simulink model "TC_SIM"  (R2025b)
settings: Solver=VariableStepAuto  StartTime=0.0  StopTime=10.0  RelTol=1e-12
values from neighbouring files (symbols this model uses):
  A = 1    [PARAMS.m]    (also in PARAMS_IDEAL_LAUNCH_TABLE.m; PID_TUNER.m)
  Cd = 1    [PARAMS.m]    (also in PARAMS_IDEAL_LAUNCH_TABLE.m; PID_TUNER.m)
  cg_f = 0.734568    [PARAMS.m]    (also in PARAMS_IDEAL_LAUNCH_TABLE.m; PID_TUNER.m)
  Cl = 3.8    [PARAMS.m]    (also in PARAMS_IDEAL_LAUNCH_TABLE.m; PID_TUNER.m)
  D = 0    [PID_TUNER.m]
  fd = 4.5    [PARAMS.m]    (also in PARAMS_IDEAL_LAUNCH_TABLE.m; PID_TUNER.m)
  gravity = 9.80665    [PARAMS.m]    (also in PARAMS_IDEAL_LAUNCH_TABLE.m; PID_TUNER.m)
  Grip_Fact = 1.0    (= 1)    [PARAMS.m]    (also in PARAMS_IDEAL_LAUNCH_TABLE.m; PID_TUNER.m)
  h_cg = 0.25273    [PARAMS.m]    (also in PARAMS_IDEAL_LAUNCH_TABLE.m; PID_TUNER.m)
  J = 0.51151    [PARAMS.m]    (also in PARAMS_IDEAL_LAUNCH_TABLE.m; PID_TUNER.m = 1.2)
  Max_Wheel_Omega = (Max_Motor_RPM * 2*pi/60) / fd    (= 162.897396853)    [PARAMS.m]    (also in PARAMS_IDEAL_LAUNCH_TABLE.m; PID_TUNER.m = 183.3)
  Mv = 285.763    [PARAMS.m]    (also in PARAMS_IDEAL_LAUNCH_TABLE.m; PID_TUNER.m)
  r = 0.203    [PARAMS.m]    (also in PARAMS_IDEAL_LAUNCH_TABLE.m; PID_TUNER.m)
  rho = 1.225    [PARAMS.m]    (also in PARAMS_IDEAL_LAUNCH_TABLE.m; PID_TUNER.m)
  Slip_Target = 0.13    [PARAMS.m]    (also in PARAMS_IDEAL_LAUNCH_TABLE.m; PID_TUNER.m)
  T_request = 150    [PARAMS.m]    (also in PARAMS_IDEAL_LAUNCH_TABLE.m; PID_TUNER.m)
  W = 1.53035    [PARAMS.m]    (also in PARAMS_IDEAL_LAUNCH_TABLE.m; PID_TUNER.m)
undefined symbols (not defined in the file or in its folder): I, N, P
libraries: slpidlib x1, simulink x1
settings Model: Creator=jacks  LastModifiedBy=jacks
settings SolverCC: ZeroCrossAlgorithm=Adaptive
settings HardwareCC: ProdHWDeviceType=AMD->x86-64 (Windows64)

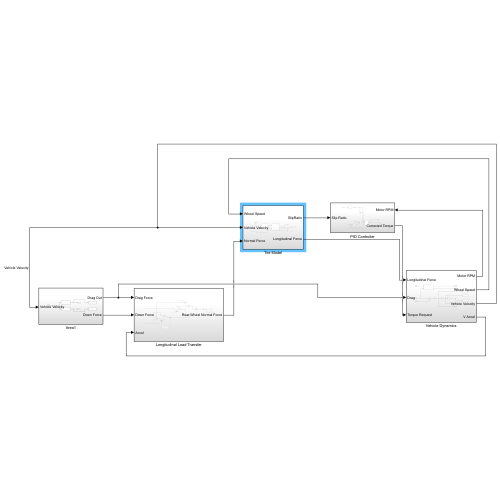
[thumbnail: Simulink's stored preview of the top-level diagram]
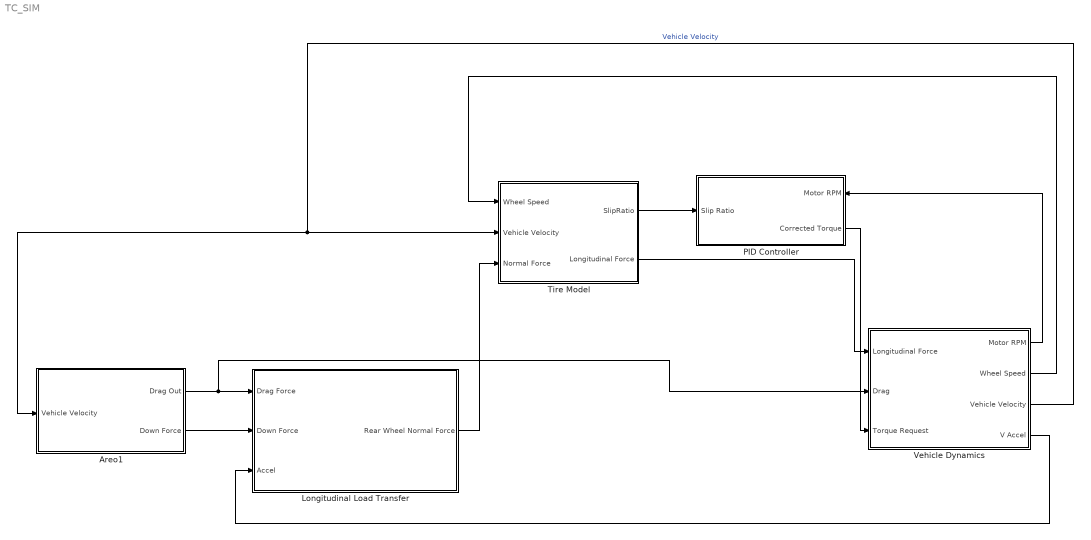
== system TC_SIM ==
  Areo1 : Subsystem
  Longitudinal Load Transfer : Subsystem
  PID Controller : Subsystem
      settings: PortSchema="{\"entries\":[{\"content\":{\"sides\":[{\"content\":{\"connectorIds\":[\"In1\"]},\"type\":\"ConnectorPlacement.EquallySpacedRectSide\",\"uuid\":\"e08c6440-e916-4e80-a3d1-0d9259b5e071\"},{\"content\":{\"connectorIds\":[\"In2\",\"Out1\"],\"side\":\"RIGHT\"},\"type\":\"ConnectorPlacement.EquallySpacedRectSide\",\"uuid\":\"5e4d30b8-f711-4660-8ae3-898fb6763926\"},{\"content\":{\"side\":\"TOP\"},\"type\":\"ConnectorPlacement.EquallySpacedRectSide\",\"uuid\":\"1af7cd33-4532-4fa2-87e1-a13d52e6b401\"}]},\"type\":\"ConnectorPlacement.EquallySpacedConnector\",\"uuid\":\"29b0d2b6-0aba-458c-9448-89d85d2daafa\"}],\"packageUris\":[\"http://schema.mathworks.com/mf0/Connector/R2020b\"],\"version\":\"1.0\"}"
  Tire Model : Subsystem
  Vehicle Dynamics : Subsystem
  wires:
  Vehicle Dynamics/3(Vehicle Velocity) -> Tire Model/2(Vehicle Velocity), Areo1/1(Vehicle Velocity)  "Vehicle Velocity"
  Tire Model/1(SlipRatio) -> PID Controller/1(Slip Ratio)
  Areo1/2(Down Force) -> Longitudinal Load Transfer/2(Down Force)
  Areo1/1(Drag Out) -> Longitudinal Load Transfer/1(Drag Force), Vehicle Dynamics/2(Drag)
  Vehicle Dynamics/4(V Accel) -> Longitudinal Load Transfer/3(Accel)
  Longitudinal Load Transfer/1(Rear Wheel Normal Force) -> Tire Model/3("Normal Force ")
  Tire Model/2(Longitudinal Force) -> Vehicle Dynamics/1(Longitudinal Force)
  Vehicle Dynamics/2(Wheel Speed) -> Tire Model/1(Wheel Speed)
  Vehicle Dynamics/1(Motor RPM) -> PID Controller/2(Motor RPM)
  PID Controller/1(Corrected Torque) -> Vehicle Dynamics/3(Torque Request)

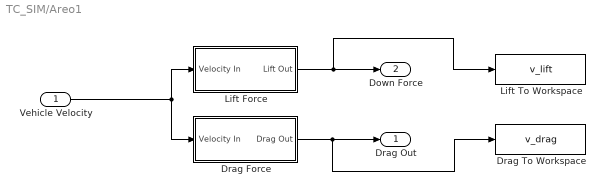
== system TC_SIM/Areo1 ==
  Vehicle Velocity : Inport
  Drag Force : Subsystem
  Drag To Workspace : ToWorkspace  VariableName=v_drag  SaveFormat=Timeseries  SampleTime=-1
  Lift Force : Subsystem
  Lift To Workspace : ToWorkspace  VariableName=v_lift  SaveFormat=Timeseries  SampleTime=-1
  Drag Out : Outport
  Down Force : Outport  Port=2
  wires:
  Lift Force/1(Lift Out) -> Lift To Workspace/1, Down Force/1
  Vehicle Velocity/1 -> Drag Force/1(Velocity In), Lift Force/1(Velocity In)
  Drag Force/1(Drag Out) -> Drag To Workspace/1, Drag Out/1

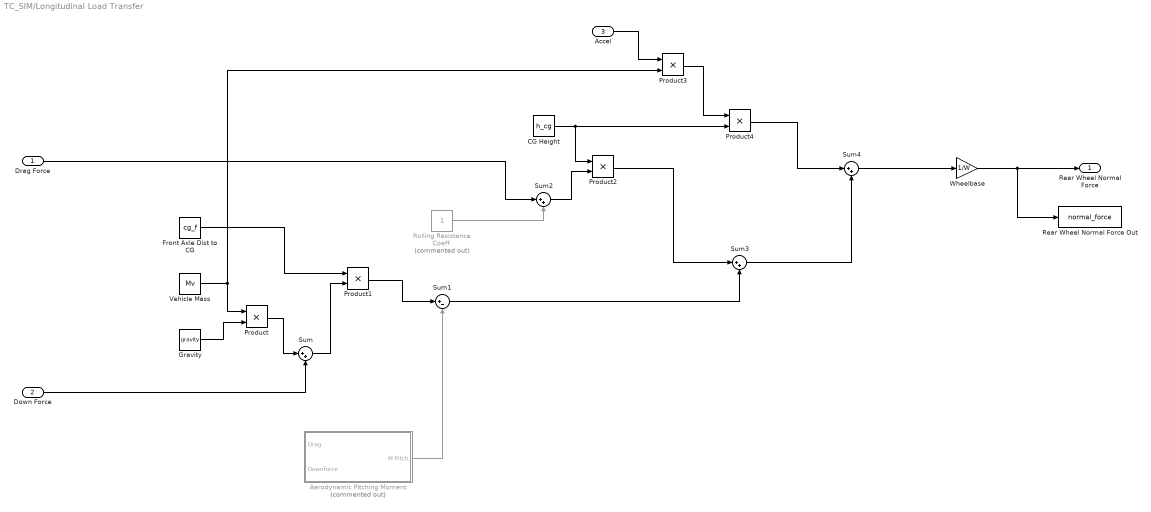
== system TC_SIM/Longitudinal Load Transfer ==
  Drag Force : Inport
  Down Force : Inport  Port=2
  Accel : Inport  Port=3
  Aerodynamic Pitching Moment : Subsystem  Commented=on
  CG Height : Constant  Value=h_cg
  Front Axle Dist to CG : Constant  Value=cg_f
  Gravity : Constant  Value=gravity
  Product{,1..4} (5 alike) : Product
  Rear Wheel Normal Force Out : ToWorkspace  VariableName=normal_force  SaveFormat=Timeseries  SampleTime=-1
  Rolling Resistance Coeff. : Constant  Commented=on
  Sum{,2..4} (4 alike) : Sum  Inputs=|++
  Sum1 : Sum  Inputs=|+-
  Vehicle Mass : Constant  Value=Mv
  Wheelbase : Gain  Gain=1/W
  Rear Wheel Normal Force : Outport
  wires:
  Vehicle Mass/1 -> Product3/2, Product/1
  Gravity/1 -> Product/2
  Down Force/1 -> Sum/2
  Product/1 -> Sum/1
  Sum/1 -> Product1/2
  Front Axle Dist to CG/1 -> Product1/1
  Product1/1 -> Sum1/1
  Drag Force/1 -> Sum2/1
  Rolling Resistance Coeff./1 -> Sum2/2
  CG Height/1 -> Product4/2, Product2/1
  Sum2/1 -> Product2/2
  Accel/1 -> Product3/1
  Product3/1 -> Product4/1
  Product2/1 -> Sum3/1
  Sum1/1 -> Sum3/2
  Product4/1 -> Sum4/1
  Sum3/1 -> Sum4/2
  Sum4/1 -> Wheelbase/1
  Wheelbase/1 -> Rear Wheel Normal Force Out/1, Rear Wheel Normal Force/1
  Aerodynamic Pitching Moment/1(M Pitch) -> Sum1/2

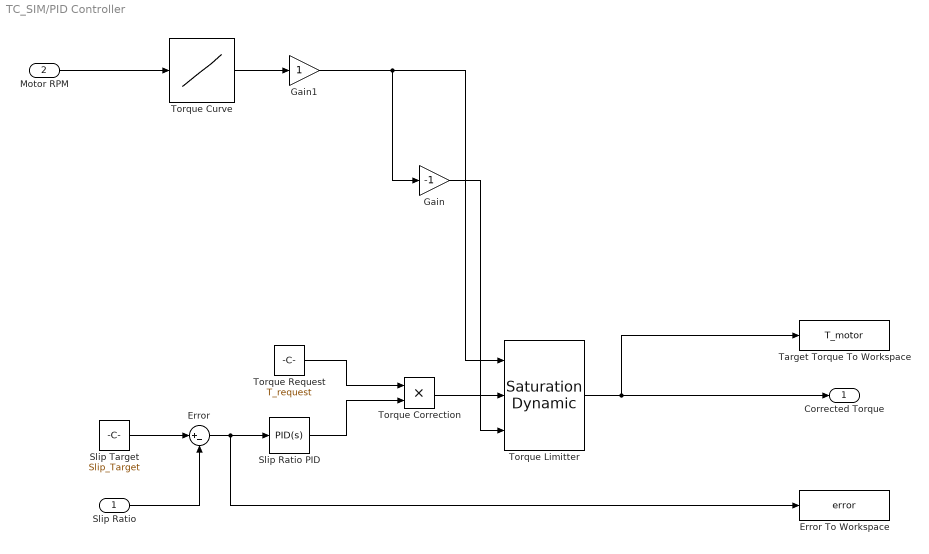
== system TC_SIM/PID Controller ==
  Slip Ratio : Inport
  Motor RPM : Inport  Port=2
  Error : Sum  Inputs=|+-
  Error To Workspace : ToWorkspace  VariableName=error  SaveFormat=Timeseries  SampleTime=-1
  Gain : Gain  Gain=-1
  Gain1 : Gain
  Slip Ratio PID : slpidlib/PID Controller  Controller=PID  Form=Parallel  TimeDomain=Continuous-time  UseExternalTs=off  SampleTime=-1  IntegratorMethod=Forward Euler  FilterMethod=Forward Euler  ControllerParametersSource=internal  P=P  I=I  UseKiTs=off  D=D  UseExternalDerivativeSource=off  N=N  UseFilter=on  TunerSelectOption=Transfer Function Based (PID Tuner App)  InitialConditionSource=internal  InitialConditionForIntegrator=0  InitialConditionForFilter=0  DifferentiatorICPrevScaledInput=0  ExternalReset=none  TrackingMode=off  Kt=1  LimitOutput=off  SatLimitsSource=internal  UpperSaturationLimit=inf  LowerSaturationLimit=-inf  LinearizeAsGain=on  AntiWindupMode=none  Kb=1  LimitIntegrator=off  UpperIntegratorSaturationLimit=inf  LowerIntegratorSaturationLimit=-inf  POutMin=[]  POutMax=[]  IOutMin=[]  IOutMax=[]  DOutMin=[]  DOutMax=[]  NOutMin=[]  NOutMax=[]  SumOutMin=[]  SumOutMax=[]  SaturationOutMin=[]  SaturationOutMax=[]  PParamMin=[]  PParamMax=[]  IParamMin=[]  IParamMax=[]  DParamMin=[]  DParamMax=[]  NParamMin=[]  NParamMax=[]  KbParamMin=[]  KbParamMax=[]  KtParamMin=[]  KtParamMax=[]  KbOutMin=[]  KbOutMax=[]  KtOutMin=[]  KtOutMax=[]  IntegratorOutMin=[]  IntegratorOutMax=[]  FilterOutMin=[]  FilterOutMax=[]  SumI1OutMin=[]  SumI1OutMax=[]  SumI2OutMin=[]  SumI2OutMax=[]  SumI3OutMin=[]  SumI3OutMax=[]  SumI4OutMin=[]  SumI4OutMax=[]  SumDOutMin=[]  SumDOutMax=[]  DifferentiatorOutMin=[]  DifferentiatorOutMax=[]  FilterDiffOutCoefMin=[]  FilterDiffOutCoefMax=[]  ReciprocalOutMin=[]  ReciprocalOutMax=[]  SumDenOutMin=[]  SumDenOutMax=[]  SumNumOutMin=[]  SumNumOutMax=[]  DivideOutMin=[]  DivideOutMax=[]  UdiffTsProdOutMin=[]  UdiffTsProdOutMax=[]  NTsProdOutMin=[]  NTsProdOutMax=[]  UintegralTsProdOutMin=[]  UintegralTsProdOutMax=[]  UngainTsProdOutMin=[]  UngainTsProdOutMax=[]  ClampingZeroOutDataTypeStr=Inherit: Inherit via back propagation  ClampingZeroOutMin=[]  ClampingZeroOutMax=[]  FilterDenConstantOutDataTypeStr=Inherit: Inherit via back propagation  FilterDenConstantOutMin=[]  FilterDenConstantOutMax=[]  PCopyOutDataTypeStr=Inherit: Inherit via back propagation  PCopyOutMin=[]  PCopyOutMax=[]  NCopyOutDataTypeStr=Inherit: Inherit via back propagation  NCopyOutMin=[]  NCopyOutMax=[]  IntegratorContinuousStateAttributes=''  IntegratorStateMustResolveToSignalObject=off  IntegratorRTWStateStorageClass=Auto  FilterContinuousStateAttributes=''  FilterStateMustResolveToSignalObject=off  FilterRTWStateStorageClass=Auto  ParallelPVariant=InternalParameters  IdealPVariant=Disabled  IVariant=InternalParameters  DVariant=InternalParameters  IntegratorVariant=Continuous  SatVariant=Disabled  AWVariant=Passthrough  PCopyVariant=Disabled  TRVariant=Disabled  FdbkBlocksVariant=Forward  IdealPFdbkVariant=Disabled  SatFdbkVariant=Disabled  DerivativeFilterVariant=ContFilter  NVariant=InternalParameters  NCopyVariant=Disabled  FilterICVariant=InternalICsFilter  IntegratorICVariant=InternalICs  ExternalResetVariant=Disabled  TRSumVariant=Passthrough  SumFdbkVariant=Disabled  SumVariant=Sum_PID  TsampFilterVariant=InternalTs  TsampNgainVariant=Passthrough  TsampIntegralVariant=Disabled_SignalSpec  ExternalSaturationOutDataTypeStr=Inherit: Same as second input  DerivativeSourceVariant=ErrorSignal  PreIntVariant=InternalPreInt
  Slip Target : Constant  Value=Slip_Target
  Target Torque To Workspace : ToWorkspace  VariableName=T_motor  SaveFormat=Timeseries  SampleTime=-1
  Torque Correction : Product
  Torque Curve : Lookup_n-D  NumberOfTableDimensions=1  BreakpointsForDimension1=[0, 500, 1000, 5000, 5400, 6000, 6998, 7000]  Table=[140, 150, 148, 148, 150, 133, 120, 0]  InternalRulePriority=Speed  RndMeth=Simplest
  Torque Limitter : simulink/Discontinuities/Saturation Dynamic  OutMin=[]  OutMax=[]  OutDataTypeStr=Inherit: Same as second input  OutDataType=fixdt(1, 16)  OutScaling=2^-10  DoSatur=off
  Torque Request : Constant  Value=T_request
  Corrected Torque : Outport
  wires:
  Slip Target/1 -> Error/1
  Error/1 -> Error To Workspace/1, Slip Ratio PID/1
  Torque Request/1 -> Torque Correction/1
  Slip Ratio/1 -> Error/2
  Torque Curve/1 -> Gain1/1
  Gain/1 -> Torque Limitter/3
  Motor RPM/1 -> Torque Curve/1
  Slip Ratio PID/1 -> Torque Correction/2
  Torque Limitter/1 -> Target Torque To Workspace/1, Corrected Torque/1
  Torque Correction/1 -> Torque Limitter/2
  Gain1/1 -> Torque Limitter/1, Gain/1

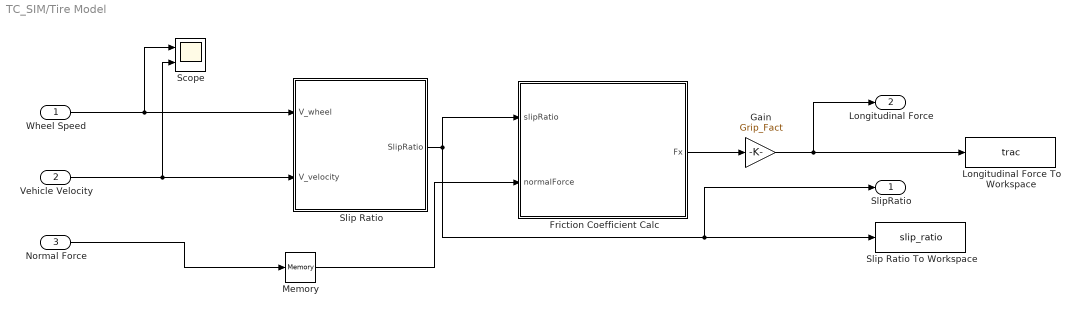
== system TC_SIM/Tire Model ==
  Wheel Speed : Inport
  Vehicle Velocity : Inport  Port=2
  "Normal Force " : Inport  Port=3
  Friction Coefficient Calc : MATLAB Function  TreatAsAtomicUnit=on
  Gain : Gain  Gain=Grip_Fact
  Longitudinal Force To Workspace : ToWorkspace  VariableName=trac  SaveFormat=Timeseries  SampleTime=-1
  Memory : Memory
  Scope : Scope  NumInputPorts=2
      settings: ActiveDisplayYMinimum=-1  ActiveDisplayYMaximum=1  DataLoggingVariableName=ScopeData2
  Slip Ratio : MATLAB Function  TreatAsAtomicUnit=on
  Slip Ratio To Workspace : ToWorkspace  VariableName=slip_ratio  SaveFormat=Timeseries  SampleTime=-1
  SlipRatio : Outport
  Longitudinal Force : Outport  Port=2
  wires:
  Slip Ratio/1(SlipRatio) -> Friction Coefficient Calc/1(slipRatio), Slip Ratio To Workspace/1, SlipRatio/1
  Vehicle Velocity/1 -> Scope/2, Slip Ratio/2(V_velocity)
  Wheel Speed/1 -> Scope/1, Slip Ratio/1(V_wheel)
  "Normal Force "/1 -> Memory/1
  Memory/1 -> Friction Coefficient Calc/2(normalForce)
  Friction Coefficient Calc/1(Fx) -> Gain/1
  Gain/1 -> Longitudinal Force To Workspace/1, Longitudinal Force/1

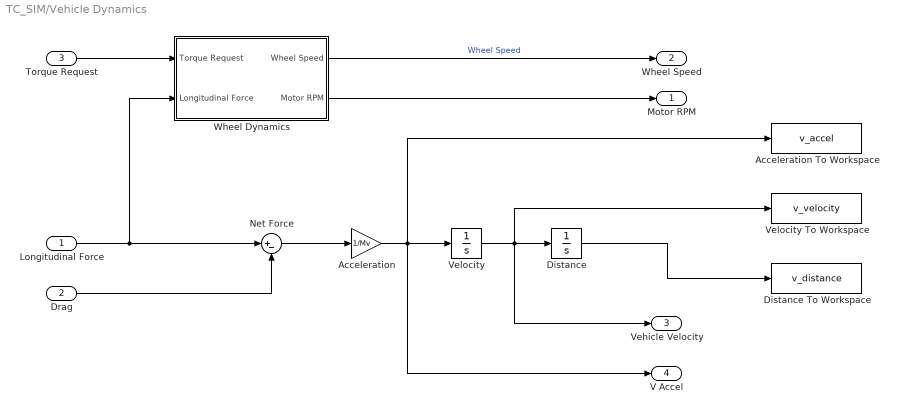
== system TC_SIM/Vehicle Dynamics ==
  Longitudinal Force : Inport
  Drag : Inport  Port=2
  Torque Request : Inport  Port=3
  Acceleration : Gain  Gain=1/Mv
  Acceleration To Workspace : ToWorkspace  VariableName=v_accel  SaveFormat=Timeseries  SampleTime=-1
  Distance : Integrator
  Distance To Workspace : ToWorkspace  VariableName=v_distance  SaveFormat=Timeseries  SampleTime=-1
  Net Force : Sum  Inputs=|+-
  "Velocity " : Integrator  InitialCondition=0.0001
  Velocity To Workspace : ToWorkspace  VariableName=v_velocity  SaveFormat=Timeseries  SampleTime=-1
  Wheel Dynamics : Subsystem
  Motor RPM : Outport
  Wheel Speed : Outport  Port=2
  Vehicle Velocity : Outport  Port=3
  V Accel : Outport  Port=4
  wires:
  "Velocity "/1 -> Vehicle Velocity/1, Velocity To Workspace/1, Distance/1
  Acceleration/1 -> V Accel/1, "Velocity "/1, Acceleration To Workspace/1
  Distance/1 -> Distance To Workspace/1
  Drag/1 -> Net Force/2
  Net Force/1 -> Acceleration/1
  Longitudinal Force/1 -> Net Force/1, Wheel Dynamics/2(Longitudinal Force)
  Torque Request/1 -> Wheel Dynamics/1(Torque Request)
  Wheel Dynamics/1(Wheel Speed) -> Wheel Speed/1  "Wheel Speed"
  Wheel Dynamics/2(Motor RPM) -> Motor RPM/1

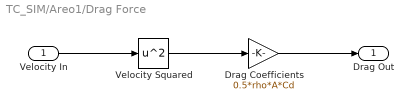
== system TC_SIM/Areo1/Drag Force ==
  Velocity In : Inport
  Drag Coefficients : Gain  Gain=0.5*rho*A*Cd
  Velocity Squared : Math  Operator=square
  Drag Out : Outport
  wires:
  Velocity In/1 -> Velocity Squared/1
  Velocity Squared/1 -> Drag Coefficients/1
  Drag Coefficients/1 -> Drag Out/1

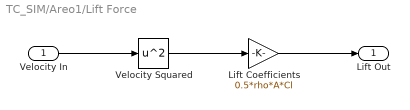
== system TC_SIM/Areo1/Lift Force ==
  Velocity In : Inport
  Lift Coefficients : Gain  Gain=0.5*rho*A*Cl
  Velocity Squared : Math  Operator=square
  Lift Out : Outport
  wires:
  Velocity Squared/1 -> Lift Coefficients/1
  Lift Coefficients/1 -> Lift Out/1
  Velocity In/1 -> Velocity Squared/1

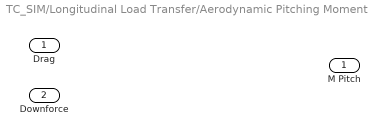
== system TC_SIM/Longitudinal Load Transfer/Aerodynamic Pitching Moment ==
  Drag : Inport
  Downforce : Inport  Port=2
  M Pitch : Outport

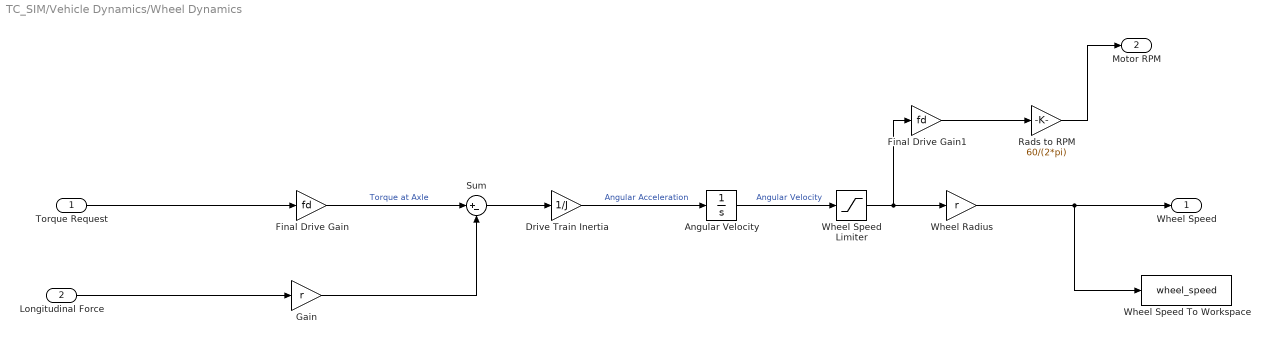
== system TC_SIM/Vehicle Dynamics/Wheel Dynamics ==
  Torque Request : Inport
  Longitudinal Force : Inport  Port=2
  Angular Velocity : Integrator
  Drive Train Inertia : Gain  Gain=1/J
  Final Drive Gain : Gain  Gain=fd
  Final Drive Gain1 : Gain  Gain=fd
  Gain : Gain  Gain=r
  Rads to RPM : Gain  Gain=60/(2*pi)
  Sum : Sum  Inputs=|+-
  Wheel Radius : Gain  Gain=r
  Wheel Speed Limiter : Saturate  UpperLimit=Max_Wheel_Omega  LowerLimit=0
  Wheel Speed To Workspace : ToWorkspace  VariableName=wheel_speed  SaveFormat=Timeseries  SampleTime=-1
  Wheel Speed : Outport
  Motor RPM : Outport  Port=2
  wires:
  Drive Train Inertia/1 -> Angular Velocity/1  "Angular Acceleration"
  Torque Request/1 -> Final Drive Gain/1
  Longitudinal Force/1 -> Gain/1
  Gain/1 -> Sum/2
  Angular Velocity/1 -> Wheel Speed Limiter/1  "Angular Velocity"
  Wheel Radius/1 -> Wheel Speed To Workspace/1, Wheel Speed/1
  Final Drive Gain1/1 -> Rads to RPM/1
  Rads to RPM/1 -> Motor RPM/1
  Wheel Speed Limiter/1 -> Final Drive Gain1/1, Wheel Radius/1
  Final Drive Gain/1 -> Sum/1  "Torque at Axle"
  Sum/1 -> Drive Train Inertia/1

== matlab function TC_SIM/Tire Model/Slip Ratio ==
  data: V_wheel input; SlipRatio output; V_velocity input
function SlipRatio = compute_slip(V_wheel, V_velocity)
    eps_val = cast(0.1, 'like', V_velocity);   
    den = max(max(abs(V_velocity), abs(V_wheel)), eps_val);  
    SlipRatio = (V_wheel - V_velocity) / den;
end

== matlab function TC_SIM/Tire Model/Friction Coefficient Calc ==
  data: slipRatio input; Fx output; normalForce input
function Fx = calculatePacejkaFx(slipRatio, normalForce)

% --- Hardcoded Model Coefficients ---
% COEFFICENTS (12 PSI FIT, 18.0x6.0-10 R20 7 in RIM)
% From 'r20_18_drive_brake_processing_aaron_comparison.m'
% Using coder.const tells Simulink these are fixed values.
B = coder.const(10.4);
C = coder.const(-1.58);
D1 = coder.const(-3.02);
D2 = coder.const(0.80);



% --- Apply the Simplified Pacejka Formula ---
% Use element-wise operators (.*, ./) to handle vector inputs

% 1. Calculate the load-dependent peak friction coefficient (mu_peak)
% The '/1000' is a scaling factor from the original data fit.
mu_peak = D1 + (D2 / 1000) .* normalForce;

% 2. Calculate the peak force (D_factor), which is mu * Fz
D_factor = mu_peak .* normalForce;

% 3. Apply the simplified Pacejka sine formula
Fx = D_factor .* sin(C * atan(B * slipRatio));

end
